simulink model "ADCS_Outline"  (R2019a)
settings: Solver=VariableStepAuto  StartTime=0.0  StopTime=duration  MaxStep=step
InitFcn:
  | SC_ODIN_INITIALIZATION
values from neighbouring files (symbols this model uses):
  A = [ v(1) v(4) v(5) v(7);        v(4) v(2) v(6) v(8);        v(5) v(6) v(3) v(9);        v(7) v(8) v(9) v(10) ]    [MagnetometerCalibration.m]    (also in SC_ODIN_INITIALIZATION.m = 0.06; test.m = asin(sin(N)/sin(n)*sin(a)))
  Amag = [0.910186583854  -0.00959593267728  0.00343590491018; -0.00959593267728  1.05471221352  0.0559849466324; 0.00343590491018  0.0559849466324  1.05528532305]    [MagnetometerBias.mat]    (also in MagnetometerCalibration.m = evecs/scale*evecs')
  argentina = [1612.36;-4182.16;-4522.83]    [SC_ODIN_INITIALIZATION.m]
  As = 0.2*0.3    (= 0.06)    [SC_ODIN_INITIALIZATION.m]
  b_mag = block.InputPort(3).Data    [MagnetometerCalibration.m]    (also in SC_ODIN_INITIALIZATION.m = [10;-15.5;-12.2]*1e-6)
  bmag = [1.00003671399e-05 -1.55007781395e-05 -1.22009762149e-05]    [MagnetometerBias.mat]    (also in MagnetometerCalibration.m = centerE)
  breakpoints = data(:,1)    [SC_ODIN_INITIALIZATION.m]
  c = 2.99792458e8    (= 299792458)    [SC_ODIN_INITIALIZATION.m]
  C_I = [0.045 0.0009 -0.00007;        0.0009 0.045 -0.00003;        -0.00007 -0.00003 0.009]    [SC_ODIN_INITIALIZATION.m]
  Cd = 2.0    (= 2)    [SC_ODIN_INITIALIZATION.m]
  controller_sample_rate = 0.5    [SC_ODIN_INITIALIZATION.m]
  D = [ 2 * x,            2 * y,            2 * z,            1 + 0 * x ]    [MagnetometerCalibration.m]    (also in SC_ODIN_INITIALIZATION.m = 0.01*[1;1;1])
  datapx = data(:,2)    [SC_ODIN_INITIALIZATION.m]
  datapy = data(:,3)    [SC_ODIN_INITIALIZATION.m]
  datapz = data(:,4)    [SC_ODIN_INITIALIZATION.m]
  datavx = data(:,5)    [SC_ODIN_INITIALIZATION.m]
  datavy = data(:,6)    [SC_ODIN_INITIALIZATION.m]
  datavz = data(:,7)    [SC_ODIN_INITIALIZATION.m]
  DCM_BT0 = eye(3)    [SC_ODIN_INITIALIZATION.m]
  G = 6.67408e-11    [SC_ODIN_INITIALIZATION.m]
  ground = [1266.06;-4295.81;4526.14]    [SC_ODIN_INITIALIZATION.m]
  I = [Ixx -Ixy -Ixz;      -Ixy Iyy -Iyz;      -Ixz -Iyz Izz]    [SC_ODIN_INITIALIZATION.m]
  invA_mag = block.InputPort(2).Data    [MagnetometerCalibration.m]    (also in SC_ODIN_INITIALIZATION.m = inv(Ellrot/scale*Ellrot'))
  JD_0 = start_day+start_fraction    [SC_ODIN_INITIALIZATION.m]
  Ks = 1367    [SC_ODIN_INITIALIZATION.m]
  L = [0.0000812 -0.0022136 -0.0225868]    [SC_ODIN_INITIALIZATION.m]
  Ls = 0.01*[-3; 3; 5]    [SC_ODIN_INITIALIZATION.m]
  M = 5.9722e24    (= 5.9722e+24)    [SC_ODIN_INITIALIZATION.m]    (also in visualisation.m = uicontrol('Style','text','String',{''},'Position',[710 100+2)
  magnetorquer_tau = 0.02    [SC_ODIN_INITIALIZATION.m]
  magnetorquer_x_saturation = 0.24    [SC_ODIN_INITIALIZATION.m]
  magnetorquer_y_saturation = 0.24    [SC_ODIN_INITIALIZATION.m]
  magnetorquer_z_saturation = 0.13    [SC_ODIN_INITIALIZATION.m]
  namibia = [5659.26;1238.85;-2659.2]    [SC_ODIN_INITIALIZATION.m]
  q = 0.6    [SC_ODIN_INITIALIZATION.m]
  radii = radii .* sgns    [MagnetometerCalibration.m]    (also in SC_ODIN_INITIALIZATION.m = [1;0.9;1.1])
  W0 = [1;0;1-1/240].*pi()/180    [SC_ODIN_INITIALIZATION.m]
  wheel_saturation = 0.23e-3    (= 0.00023)    [SC_ODIN_INITIALIZATION.m]
  wheel_tau = 2    [SC_ODIN_INITIALIZATION.m]
undefined symbols (not defined in the file or in its folder): DiscIntNeverNeededParam, nut80, sun_sensors
libraries: dspmathops x94, vrlib x70, dspsrcs4 x21, realtime_pacer_lib x1, dspsolvers x1, dspinverses x1
(part 5 of 6)

== matlab function ADCS_Outline/Sun/MATLAB Function2 ==
  data: ddpsi input; ddeps input; reci input; nut80 input; rteme output; ttt input
% ----------------------------------------------------------------------------
%
%                           function eci2teme
%
%  this function transforms a vector from the mean equator mean equinox (j2000) 
%    system (eci), to the true equator mean equinox (teme) system.
%
%  author        : david vallado                  719-573-2600   30 oct 2017
%
%  inputs          description                    range / units
%    reci        - position vector eci            km
%    veci        - velocity vector eci            km/s
%    aeci        - acceleration vector eci        km/s2
%    ttt         - julian centuries of tt         centuries
%    ddpsi       - delta psi correction to gcrf   rad
%    ddeps       - delta eps correction to gcrf   rad
%
%  outputs       :
%    rteme       - position vector of date
%                    true equator, mean equinox   km
%    vteme       - velocity vector of date
%                    true equator, mean equinox   km/s
%    ateme       - acceleration vector of date
%                    true equator, mean equinox   km/s2
%
%  locals        :
%    prec        - matrix for eci - mod
%    nutteme     - matrix for mod - teme - an approximation for nutation
%    eqe         - rotation for equation of equinoxes (geometric terms only)
%    tm          - combined matrix for teme2eci
%
%  coupling      :
%   precess      - rotation for precession        eci - mod
%   nutation     - rotation for nutation          eci - tod
%
%  references    :
%    vallado       2013, 231-233
%
% [reci, veci, aeci] = teme2eci  ( rteme, vteme, ateme, ttt, ddpsi, ddeps);
% ----------------------------------------------------------------------------

function rteme  = eci2teme  (ddpsi, ddeps, reci, nut80, ttt)

        prec = zeros(3,3);
        [prec,psia, wa, ea, xa] = precess ( ttt );

        [deltapsi, trueeps, meaneps, omega, nut] = nutation  (ttt, ddpsi, ddeps, nut80);
        
        % ------------------------ find eqeg ----------------------
        % rotate teme through just geometric terms 
        eqeg = deltapsi* cos(meaneps);

        eqeg = rem (eqeg, 2.0*pi);

        eqe = zeros(3,3);
        eqe(1,1) =  cos(eqeg);
        eqe(1,2) =  sin(eqeg);
        eqe(1,3) =  0.0;
        eqe(2,1) = -sin(eqeg);
        eqe(2,2) =  cos(eqeg);
        eqe(2,3) =  0.0;
        eqe(3,1) =  0.0;
        eqe(3,2) =  0.0;
        eqe(3,3) =  1.0;

        tm = eqe * nut' * prec';
        
        rteme = tm * reci;
        

%�
% ----------------------------------------------------------------------------
%
%                           function precess
%
%  this function calulates the transformation matrix that accounts for the effects
%    of precession. both the 1980 and 2000 theories are handled. note that the 
%    required parameters differ a little. 
%
%  author        : david vallado                  719-573-2600   25 jun 2002
%
%  revisions
%    vallado     - consolidate with iau 2000                     14 feb 2005
%
%  inputs          description                    range / units
%    ttt         - julian centuries of tt
%    opt         - method option                  '01', '02', '96', '80'
%
%  outputs       :
%    prec        - transformation matrix for mod - j2000 (80 only)
%    psia        - cannonical precession angle    rad    (00 only)
%    wa          - cannonical precession angle    rad    (00 only)
%    ea          - cannonical precession angle    rad    (00 only)
%    xa          - cannonical precession angle    rad    (00 only)
%
%  locals        :
%    ttt2        - ttt squared
%    ttt3        - ttt cubed
%    zeta        - precession angle               rad
%    z           - precession angle               rad
%    theta       - precession angle               rad
%    oblo        - obliquity value at j2000 epoch "%
%
%  coupling      :
%    none        -
%
%  references    :
%    vallado       2004, 214-216, 219-221
%
% [prec,psia,wa,ea,xa] = precess ( ttt, opt );
% ----------------------------------------------------------------------------

function [prec,psia,wa,ea,xa] = precess ( ttt );

       % sethelp;
        
        % " to rad
        convrt = pi / (180.0*3600.0);
        ttt2= ttt * ttt;
        ttt3= ttt2 * ttt;

        % ------------------- fk4 b1950 precession angles --------------------
%         if (opt == '50')
% 
%             % ---- Seidelmann pg 107             
%             % for these calls, ttt will come in with the current jd
% %            t1= 0.0; %(ttt - 2433282.42345905)/365242.198782;  % set start as B1850, 0.0 to simplify
% %            t2= (ttt - 2396758.203)/365242.198782;  % uses B1850
% %            ttt = t2 - t1;
% %            ttt2 = ttt * ttt;
% %            ttt3 = ttt * ttt2;
% %            fprintf(1,'50prec %15.9f  \n',ttt);
%             % exp supp 61 pg 38
% %            psia = 50.3708 + 0.0050 * ttt;
% %            wa = 0.0;
% %            ea = 0.0;
% %            xa = 0.1247 - 0.0188 * ttt;
% %            zeta =  (23035.545 + 139.720*t1 + 0.060 *t1*t1)*ttt + (30.240-0.270*t1)*ttt2 + 17.995*ttt3; % "
% %            theta=  (20051.12 - 85.29*t1 - 0.37 *t1*t1)*ttt + (-42.65-0.37*t1)*ttt2 - 41.80*ttt3;
% %            z    =  (23035.545 + 139.720*t1 + 0.060 *t1*t1)*ttt + (109.480+0.390*t1)*ttt2 + 18.325*ttt3;
% 
%             % ---- Newcomb Exp Supp 61 approach, but see GTDS pg 3-17
%             % Exp Supp 61 says use 1900? but gtds says use 1950. 
%             % for these calls, ttt will come in with the current jd
%             t1= 0.0; %(ttt - 2415020.31352)/36524.2198782;  % set start as B1900, 0.0 to simplify
% %            t2= (ttt - 2415020.31352)/36525;  % uses B1900   
%             t2= (ttt - 2433282.42345905)/36525;  % uses B1950  
% %            ttt = t2 - t1;
% %            ttt2 = ttt * ttt;
% %            ttt3 = ttt * ttt2;
%             % exp supp 61 pg 38
%             psia = 50.3708 + 0.0050 * ttt;
%             wa = 0.0; % not sure which one is which...
%             ea = 84428.26 -   46.845*ttt - 0.00059*ttt2 + 0.00181*ttt3;
%             xa = 0.1247 - 0.0188 * ttt;
%            fprintf(1,'50prec %15.9f  \n',ttt);
%            % seems like Exp supp 61 is ok with 1900 as epoch, and Seidlemann is ok with listed measr,  
% %            zeta =  (2304.25 + 1.396*t1)*ttt + 0.302*ttt2 + 0.018*ttt3; % "
% %            theta=  (2004.682 - 0.853*t1)*ttt -0.426*ttt2 - 0.042*ttt3;
% %            z    =  (2304.25 + 1.396*t1)*ttt + 1.093*ttt2 + 0.018*ttt3;
%             % GTDS pg 3-17 using days from 1950 - avoids long rpecession
%             % constants...
%             zeta =  2304.9969*ttt + 0.302*ttt2 + 0.01808*ttt3; % "
%             theta=  2004.2980*ttt -0.425936*ttt2 - 0.0416*ttt3;
%             z    =  2304.9969*ttt + 1.092999*ttt2 + 0.0192*ttt3;
%             
% 
%             % tp-008 36-45
%             % ttt is tropical centruies from 1950 36524.22 days
%             prec = zeros(3,3);
%             prec(1,1) =  1.0 - 2.9696e-4 * ttt2 - 1.3e-7 * ttt3;
%             prec(1,2) =  2.234941e-2 * ttt + 6.76e-6 * ttt2 - 2.21e-6 * ttt3;
%             prec(1,3) =  9.7169e-3 * ttt - 2.07e-6 * ttt2 - 9.6e-7 * ttt3;
%             prec(2,1) =  -prec(1,2);
%             prec(2,2) =  1.0 - 2.4975e-4 * ttt2 - 1.5e-7 * ttt3;
%             prec(2,3) =  - 1.0858e-4 * ttt2;
%             prec(3,1) =  -prec(1,3);
%             prec(3,2) =  prec(2,3);
%             prec(3,3) =  1.0 - 4.721e-5 * ttt2;
%  
%             
%            % pass these back out for testing
%            psia = zeta;
%            wa = theta;
%            ea = z;
%         % ------------------- iau 76 precession angles --------------------
%         else
%           if (opt == '80')
%     fprintf(1,'80prec %15.9f  \n',ttt);
            psia =             5038.7784*ttt - 1.07259*ttt2 - 0.001147*ttt3; % "
            wa   = 84381.448                 + 0.05127*ttt2 - 0.007726*ttt3;
            ea   = 84381.448 -   46.8150*ttt - 0.00059*ttt2 + 0.001813*ttt3;
            xa   =               10.5526*ttt - 2.38064*ttt2 - 0.001125*ttt3;
            zeta =             2306.2181*ttt + 0.30188*ttt2 + 0.017998*ttt3; % "
            theta=             2004.3109*ttt - 0.42665*ttt2 - 0.041833*ttt3;
            z    =             2306.2181*ttt + 1.09468*ttt2 + 0.018203*ttt3;
          % ------------------ iau 03 precession angles -------------------
%           else
%             oblo =  84381.406; % "
%             psia =  (((( -0.0000000951 * ttt + 0.000132851 ) * ttt - 0.00114045 ) * ttt - 1.0790069 ) * ttt + 5038.481507 ) * ttt; % "
%             wa   =  ((((  0.0000003337 * ttt - 0.000000467 ) * ttt - 0.00772503 ) * ttt + 0.0512623 ) * ttt -    0.025754 ) * ttt + oblo;
%             ea   =  (((( -0.0000000434 * ttt - 0.000000576 ) * ttt + 0.00200340 ) * ttt - 0.0001831 ) * ttt -   46.836769 ) * ttt + oblo;
%             xa   =  (((( - 0.0000000560 * ttt + 0.000170663 ) * ttt - 0.00121197 ) * ttt - 2.3814292 ) * ttt +   10.556403 ) * ttt;
% 
%             zeta =  (((( - 0.0000003173 * ttt - 0.000005971 ) * ttt + 0.01801828 ) * ttt + 0.2988499 ) * ttt + 2306.083227 ) * ttt + 2.650545; % "
%             theta=  (((( - 0.0000001274 * ttt - 0.000007089 ) * ttt - 0.04182264 ) * ttt - 0.4294934 ) * ttt + 2004.191903 ) * ttt;
%             z    =  ((((   0.0000002904 * ttt - 0.000028596 ) * ttt + 0.01826837 ) * ttt + 1.0927348 ) * ttt + 2306.077181 ) * ttt - 2.650545;
%           end;
%         end;
        
        % convert units to rad
        psia = psia  * convrt; % rad
        wa   = wa    * convrt;
        ea   = ea    * convrt;
        xa   = xa    * convrt;
        zeta = zeta  * convrt; 
        theta= theta * convrt;
        z    = z     * convrt;
%iauhelp='y';         
%fprintf(1,'pr %11.7f  %11.7f  %11.7fdeg \n',zeta*180/pi,theta*180/pi,z*180/pi );
%         if (iauhelp == 'y')
%             fprintf(1,'pr %11.7f  %11.7f  %11.7f %11.7fdeg \n',psia*180/pi,wa*180/pi,ea*180/pi,xa*180/pi );
%             fprintf(1,'pr %11.7f  %11.7f  %11.7fdeg \n',zeta*180/pi,theta*180/pi,z*180/pi );
%         end;
% 
%         if (strcmp(opt,'80')==1) % || (strcmp(opt,'50') == 1)
            coszeta  = cos(zeta);
            sinzeta  = sin(zeta);
            costheta = cos(theta);
            sintheta = sin(theta);
            cosz     = cos(z);
            sinz     = sin(z);

            % ----------------- form matrix  mod to j2000 -----------------
            prec = zeros(3,3);
            prec(1,1) =  coszeta * costheta * cosz - sinzeta * sinz;
            prec(1,2) =  coszeta * costheta * sinz + sinzeta * cosz;
            prec(1,3) =  coszeta * sintheta;
            prec(2,1) = -sinzeta * costheta * cosz - coszeta * sinz;
            prec(2,2) = -sinzeta * costheta * sinz + coszeta * cosz;
            prec(2,3) = -sinzeta * sintheta;
            prec(3,1) = -sintheta * cosz;
            prec(3,2) = -sintheta * sinz;
            prec(3,3) =  costheta;

            % ----------------- do rotations instead ----------------------
            % p1 = rot3mat( z );
            % p2 = rot2mat( -theta );
            % p3 = rot3mat( zeta );
            % prec = p3*p2*p1;
%         elseif (strcmp(opt,'50') ~= 1)
%             oblo = oblo * convrt; % " to rad
%             a4  = rot3mat(-xa);
%             a5  = rot1mat(wa);
%             a6  = rot3mat(psia);
%             a7  = rot1mat(-oblo);
%             prec = a7*a6*a5*a4;
%            % prec = zeros(3);
%         end;



% ----------------------------------------------------------------------------
%
%                           function nutation
%
%  this function calulates the transformation matrix that accounts for the
%    effects of nutation.
%
%  author        : david vallado                  719-573-2600   27 jun 2002
%
%  revisions
%    vallado     - consolidate with iau 2000                     14 feb 2005
%
%  inputs          description                    range / units
%    ttt         - julian centuries of tt
%    ddpsi       - delta psi correction to gcrf   rad
%    ddeps       - delta eps correction to gcrf   rad
%
%  outputs       :
%    deltapsi    - nutation angle                 rad
%    trueeps     - true obliquity of the ecliptic rad
%    meaneps     - mean obliquity of the ecliptic rad
%    omega       -                                rad
%    nut         - transformation matrix for tod - mod
%
%  locals        :
%    iar80       - integers for fk5 1980
%    rar80       - reals for fk5 1980
%    ttt2        - ttt squared
%    ttt3        - ttt cubed
%    l           -                                rad
%    ll          -                                rad
%    f           -                                rad
%    d           -                                rad
%    deltaeps    - change in obliquity            rad
%
%  coupling      :
%    fundarg     - find fundamental arguments
%
%  references    :
%    vallado       2013, 224-226
%
% [deltapsi, trueeps, meaneps, omega,nut] = nutation  (ttt, ddpsi, ddeps );
% ----------------------------------------------------------------------------

function [deltapsi, trueeps, meaneps, omega,nut] = nutation  (ttt, ddpsi, ddeps , nut80);

        deg2rad = pi/180.0;

        [iar80,rar80] =  iau80in(nut80);  % coeff in deg

        % ---- determine coefficients for iau 1980 nutation theory ----
        ttt2= ttt*ttt;
        ttt3= ttt2*ttt;

        meaneps = -46.8150 *ttt - 0.00059 *ttt2 + 0.001813 *ttt3 + 84381.448;
        meaneps = rem( meaneps/3600.0, 360.0 );
        meaneps = meaneps * deg2rad;

        [ l, l1, f, d, omega, ...
          lonmer, lonven, lonear, lonmar, lonjup, lonsat, lonurn, lonnep, precrate ...
        ] = fundarg( ttt, '80' );
%fprintf(1,'nut del arg %11.7f  %11.7f  %11.7f  %11.7f  %11.7f  \n',l*180/pi,l1*180/pi,f*180/pi,d*180/pi,omega*180/pi );

        deltapsi= 0.0;
        deltaeps= 0.0;
        for i= 106:-1: 1
            tempval= iar80(i,1)*l + iar80(i,2)*l1 + iar80(i,3)*f + ...
                     iar80(i,4)*d + iar80(i,5)*omega;
            deltapsi= deltapsi + (rar80(i,1)+rar80(i,2)*ttt) * sin( tempval );
            deltaeps= deltaeps + (rar80(i,3)+rar80(i,4)*ttt) * cos( tempval );
        end

        % --------------- find nutation parameters --------------------
        deltapsi = rem( deltapsi + ddpsi, 2.0 * pi );
        deltaeps = rem( deltaeps + ddeps, 2.0 * pi );
        trueeps  = meaneps + deltaeps;

%fprintf(1,'meaneps %11.7f dp  %11.7f de  %11.7f te  %11.7f  ttt  %11.7f \n',meaneps*180/pi,deltapsi*180/pi,deltaeps*180/pi,trueeps*180/pi, ttt );

        cospsi  = cos(deltapsi);
        sinpsi  = sin(deltapsi);
        coseps  = cos(meaneps);
        sineps  = sin(meaneps);
        costrueeps = cos(trueeps);
        sintrueeps = sin(trueeps);
        
        nut = zeros(3,3);
        nut(1,1) =  cospsi;
        nut(1,2) =  costrueeps * sinpsi;
        nut(1,3) =  sintrueeps * sinpsi;
        nut(2,1) = -coseps * sinpsi;
        nut(2,2) =  costrueeps * coseps * cospsi + sintrueeps * sineps;
        nut(2,3) =  sintrueeps * coseps * cospsi - sineps * costrueeps;
        nut(3,1) = -sineps * sinpsi;
        nut(3,2) =  costrueeps * sineps * cospsi - sintrueeps * coseps;
        nut(3,3) =  sintrueeps * sineps * cospsi + costrueeps * coseps;

      %   n1 = rot1mat( trueeps );
      %   n2 = rot3mat( deltapsi );
      %   n3 = rot1mat( -meaneps );
      %   nut = n3*n2*n1

%�
% ----------------------------------------------------------------------------
%
%                           function fundarg
%
%  this function calulates the delauany variables and planetary values for
%  several theories.
%
%  author        : david vallado                  719-573-2600   16 jul 2004
%
%  revisions
%    vallado     - consolidate with iau 2000                     14 feb 2005
%
%  inputs          description                    range / units
%    ttt         - julian centuries of tt
%    opt         - method option                  '10', '02', '96', '80'
%
%  outputs       :
%    l           - delaunay element               rad
%    ll          - delaunay element               rad
%    f           - delaunay element               rad
%    d           - delaunay element               rad
%    omega       - delaunay element               rad
%    planetary longitudes                         rad
%
%  locals        :
%    ttt2,ttt3,  - powers of ttt
%
%  coupling      :
%    none        -
%
%  references    :
%    vallado       2004, 212-214
%
% [ l, l1, f, d, omega, ...
%   lonmer, lonven, lonear, lonmar, lonjup, lonsat, lonurn, lonnep, precrate ...
% ] = fundarg( ttt, opt );
% ----------------------------------------------------------------------------

function [ l, l1, f, d, omega, ...
           lonmer, lonven, lonear, lonmar, lonjup, lonsat, lonurn, lonnep, precrate ...
         ] = fundarg( ttt, opt )

        %sethelp;

        deg2rad = pi/180.0;

        % ---- determine coefficients for iau 2000 nutation theory ----
        ttt2 = ttt*ttt;
        ttt3 = ttt2*ttt;
        ttt4 = ttt2*ttt2;

        % ---- iau 2010 theory
        if opt == '10'
            % ------ form the delaunay fundamental arguments in deg
            l    =  134.96340251  + ( 1717915923.2178 *ttt + ...
                     31.8792 *ttt2 + 0.051635 *ttt3 - 0.00024470 *ttt4 ) / 3600.0;
            l1   =  357.52910918  + (  129596581.0481 *ttt - ...
                      0.5532 *ttt2 - 0.000136 *ttt3 - 0.00001149*ttt4 )  / 3600.0;
            f    =   93.27209062  + ( 1739527262.8478 *ttt - ...
                     12.7512 *ttt2 + 0.001037 *ttt3 + 0.00000417*ttt4 )  / 3600.0;
            d    =  297.85019547  + ( 1602961601.2090 *ttt - ...
                      6.3706 *ttt2 + 0.006593 *ttt3 - 0.00003169*ttt4 )  / 3600.0;
            omega=  125.04455501  + (   -6962890.5431 *ttt + ...
                      7.4722 *ttt2 + 0.007702 *ttt3 - 0.00005939*ttt4 )  / 3600.0;

            % ------ form the planetary arguments in deg
            lonmer  = 252.250905494  + 149472.6746358  *ttt;
            lonven  = 181.979800853  +  58517.8156748  *ttt;
            lonear  = 100.466448494  +  35999.3728521  *ttt;
            lonmar  = 355.433274605  +  19140.299314   *ttt;
            lonjup  =  34.351483900  +   3034.90567464 *ttt;
            lonsat  =  50.0774713998 +   1222.11379404 *ttt;
            lonurn  = 314.055005137  +    428.466998313*ttt;
            lonnep  = 304.348665499  +    218.486200208*ttt;
            precrate=   1.39697137214*ttt + 0.0003086*ttt2;
         end;

        % ---- iau 2000b theory
        if opt == '02'
            % ------ form the delaunay fundamental arguments in deg
            l    =  134.96340251  + ( 1717915923.2178 *ttt ) / 3600.0;
            l1   =  357.52910918  + (  129596581.0481 *ttt ) / 3600.0;
            f    =   93.27209062  + ( 1739527262.8478 *ttt ) / 3600.0;
            d    =  297.85019547  + ( 1602961601.2090 *ttt ) / 3600.0;
            omega=  125.04455501  + (   -6962890.5431 *ttt ) / 3600.0;

            % ------ form the planetary arguments in deg
            lonmer  = 0.0;
            lonven  = 0.0;
            lonear  = 0.0;
            lonmar  = 0.0;
            lonjup  = 0.0;
            lonsat  = 0.0;
            lonurn  = 0.0;
            lonnep  = 0.0;
            precrate= 0.0;
         end;   

        % ---- iau 1996 theory
        if opt == '96'
            l    =  134.96340251  + ( 1717915923.2178 *ttt + ...
                     31.8792 *ttt2 + 0.051635 *ttt3 - 0.00024470 *ttt4 ) / 3600.0;
            l1   =  357.52910918  + (  129596581.0481 *ttt - ...
                      0.5532 *ttt2 - 0.000136 *ttt3 - 0.00001149*ttt4 )  / 3600.0;
            f    =   93.27209062  + ( 1739527262.8478 *ttt - ...
                     12.7512 *ttt2 + 0.001037 *ttt3 + 0.00000417*ttt4 )  / 3600.0;
            d    =  297.85019547  + ( 1602961601.2090 *ttt - ...
                      6.3706 *ttt2 + 0.006593 *ttt3 - 0.00003169*ttt4 )  / 3600.0;
            omega=  125.04455501  + (   -6962890.2665 *ttt + ...
                      7.4722 *ttt2 + 0.007702 *ttt3 - 0.00005939*ttt4 )  / 3600.0;
            % ------ form the planetary arguments in deg
            lonmer  = 0.0;
            lonven  = 181.979800853  +  58517.8156748  *ttt;   % deg
            lonear  = 100.466448494  +  35999.3728521  *ttt;
            lonmar  = 355.433274605  +  19140.299314   *ttt;
            lonjup  =  34.351483900  +   3034.90567464 *ttt;
            lonsat  =  50.0774713998 +   1222.11379404 *ttt;
            lonurn  = 0.0;
            lonnep  = 0.0;
            precrate=   1.39697137214*ttt + 0.0003086*ttt2;
         end;   

         % ---- iau 1980 theory
        if opt == '80'
            l = ((((0.064) * ttt + 31.310) * ttt + 1717915922.6330) * ttt) / 3600.0 + 134.96298139;
    		l1 = ((((-0.012) * ttt - 0.577) * ttt + 129596581.2240) * ttt) / 3600.0 + 357.52772333;
    		f = ((((0.011) * ttt - 13.257) * ttt + 1739527263.1370) * ttt) / 3600.0 + 93.27191028;
	    	d = ((((0.019) * ttt - 6.891) * ttt + 1602961601.3280) * ttt) / 3600.0 + 297.85036306;
    		omega = ((((0.008) * ttt + 7.455) * ttt - 6962890.5390) * ttt) / 3600.0 + 125.04452222;
                  
            % ------ form the planetary arguments in deg
            lonmer  = 252.3 + 149472.0 *ttt;
            lonven  = 179.9 +  58517.8 *ttt;   % deg
            lonear  =  98.4 +  35999.4 *ttt;
            lonmar  = 353.3 +  19140.3 *ttt;
            lonjup  =  32.3 +   3034.9 *ttt;
            lonsat  =  48.0 +   1222.1 *ttt;
            lonurn  =   0.0;
            lonnep  =   0.0;
            precrate=   0.0;
         end;   

        % ---- convert units to rad
        l    = rem( l,360.0  )     * deg2rad; % rad
        l1   = rem( l1,360.0  )    * deg2rad;
        f    = rem( f,360.0  )     * deg2rad;
        d    = rem( d,360.0  )     * deg2rad;
        omega= rem( omega,360.0  ) * deg2rad;

        lonmer= rem( lonmer,360.0 ) * deg2rad;  % rad
        lonven= rem( lonven,360.0 ) * deg2rad;
        lonear= rem( lonear,360.0 ) * deg2rad;
        lonmar= rem( lonmar,360.0 ) * deg2rad;
        lonjup= rem( lonjup,360.0 ) * deg2rad;
        lonsat= rem( lonsat,360.0 ) * deg2rad;
        lonurn= rem( lonurn,360.0 ) * deg2rad;
        lonnep= rem( lonnep,360.0 ) * deg2rad;
        precrate= rem( precrate,360.0 ) * deg2rad;
%iauhelp='y';
%         if iauhelp == 'y'
%             fprintf(1,'fa %11.7f  %11.7f  %11.7f  %11.7f  %11.7f deg \n',l*180/pi,l1*180/pi,f*180/pi,d*180/pi,omega*180/pi );
%             fprintf(1,'fa %11.7f  %11.7f  %11.7f  %11.7f deg \n',lonmer*180/pi,lonven*180/pi,lonear*180/pi,lonmar*180/pi );
%             fprintf(1,'fa %11.7f  %11.7f  %11.7f  %11.7f deg \n',lonjup*180/pi,lonsat*180/pi,lonurn*180/pi,lonnep*180/pi );
%             fprintf(1,'fa %11.7f  \n',precrate*180/pi );
%           end;

function [iar80,rar80] = iau80in(nut80);

       % ------------------------  implementation   -------------------
       % 0.0001" to rad
       convrt= 0.0001 * pi / (180*3600.0);

       %load nut80.dat;

       iar80 = nut80(:,1:5);
       rar80 = nut80(:,6:9);

       for i=1:106
           for j=1:4
               rar80(i,j)= rar80(i,j) * convrt;
           end
       end

== matlab function ADCS_Outline/S//C Kinematics/Skewed/MATLAB Function ==
  data: u input; y output
function y = fcn(u)
y = [0 -u(3) u(2); ...
     u(3) 0 -u(1); ...
    -u(2) u(1) 0];

== matlab function ADCS_Outline/Momentum Control/Momentum Bias/Rotation/     ==
  data: qa input; q output; qb input
function q = Quatmultiply(qa,qb)

q4 = qa(4)*qb(4) - qa(1)*qb(1) - qa(2)*qb(2) - qa(3)*qb(3);
q1 = qa(4)*qb(1) + qa(1)*qb(4) + qa(2)*qb(3) - qa(3)*qb(2);
q2 = qa(4)*qb(2) - qa(1)*qb(3) + qa(2)*qb(4) + qa(3)*qb(1);
q3 = qa(4)*qb(3) + qa(1)*qb(2) - qa(2)*qb(1) + qa(3)*qb(4);

q = [q1 q2 q3 q4];

== matlab function ADCS_Outline/Reaction Wheels/MATLAB Function ==
  data: Ti input; Tw output; Lw input
function Tw = saturation_rw(Ti,Lw)

sat1 = abs(Lw(1))/1.77e-3;
sat2 = abs(Lw(2))/1.77e-3;
sat3 = abs(Lw(3))/1.77e-3;

if sat1>1 && Ti(1)*Lw(1)>0
    T1 = 0;
else 
    T1 = Ti(1);
end

if sat2>1 && Ti(2)*Lw(2)>0
    T2 = 0;
else 
    T2 = Ti(2);
end

if sat3>1 && Ti(3)*Lw(3)>0
    T3 = 0;
else 
    T3 = Ti(3);
end

Tw = [T1;T2;T3];

== matlab function ADCS_Outline/Toolbox/No Control fast STK attitude recoding/Mode Selector ==
  data: P input; A input; N input; G input; Mode output
function Mode  = Selector(P,A,N,G)

        if dot(P,A)/(norm(P)*norm(A)) > 0.96 %In range of Argentina
           Mode = 3; %Imaging Argentina
        elseif dot(P,N)/(norm(P)*norm(N)) > 0.96 %In range of Namibia
           Mode = 4; %Imaging Namibia 
        elseif dot(P,G)/(norm(P)*norm(G)) > 0.91 %In range of ground
           Mode = 2; %Ground
        else
           Mode = 5; %Nadir  
        end

end

== matlab function ADCS_Outline/VISUALISATION/MATLAB Function2 ==
  data: DCM input; yaw output; pitch output; roll output
function [yaw, pitch, roll] = DCM2euler(DCM)

yaw = atan2(DCM(2,1),DCM(1,1));
pitch = asin(min(1, max(-1, -DCM(3,1))));
roll = atan2(DCM(3,2),DCM(3,3));

end

== matlab function ADCS_Outline/Momentum Control/Momentum Bias/Rotation/    1 ==
  data: qa input; q output; qb input
function q = Quatmultiply(qa,qb)

q4 = qa(4)*qb(4) - qa(1)*qb(1) - qa(2)*qb(2) - qa(3)*qb(3);
q1 = qa(4)*qb(1) + qa(1)*qb(4) + qa(2)*qb(3) - qa(3)*qb(2);
q2 = qa(4)*qb(2) - qa(1)*qb(3) + qa(2)*qb(4) + qa(3)*qb(1);
q3 = qa(4)*qb(3) + qa(1)*qb(2) - qa(2)*qb(1) + qa(3)*qb(4);

q = [q1 q2 q3 q4];

== matlab function ADCS_Outline/Toolbox/No Control fast STK attitude recoding/Perfect DCM1/Mode Selection ==
  data: Mode input; DCM_EF input; DCM_FS input; DCM_ETarget output; DCM_FG input; DCM_FA input; DCM_FN input; DCM_FZ input
function DCM_ETarget   = fcn(Mode,DCM_EF,DCM_FS,DCM_FG, DCM_FA, DCM_FN, DCM_FZ)

switch Mode
    case 1
      DCM_ETarget = DCM_EF*DCM_FS;
    case 2
      DCM_ETarget = DCM_EF*DCM_FG;
    case 3
      DCM_ETarget = DCM_EF*DCM_FA;
    case 4
      DCM_ETarget = DCM_EF*DCM_FN;
    case 5
      DCM_ETarget = DCM_EF*DCM_FZ;
    otherwise 
      DCM_ETarget = eye(3);
end

== matlab function ADCS_Outline/Momentum Control/Switch ==
  data: CM output; Mode input; Eclipse input; Bdot input; M output; Nominal input
function [CM,M] = fcn(Mode,Eclipse,Bdot,Nominal)

persistent pause

switch Mode
    
    case 2 %ground
        M = [0;0;0];
        CM = [0;0;0];
    case 3 %imagingA
        M = [0;0;0];
        CM = [0;0;0];
    case 4 %imgaing N
        M = [0;0;0];
        CM = [0;0;0];
    case 6 %detumbling
        M = Bdot;
        CM = Bdot;
    case 7 %OFF
        M = [0;0;0];
        CM = [0;0;0];
    case 8 %calibration
        M = [0;0;0];
        CM = [0;0;0];
    otherwise
        M = Nominal;
        CM = Nominal;
        
end

if isempty(pause)
    pause = 1;
elseif pause >=1%stops magnetorquers to get a reading
    pause = 0;
    M = [0;0;0];
    CM = Nominal;
elseif ismember(Mode,[1 5 6])
    pause = pause + 1;
end

if (Eclipse == 1) && (Mode~=6)
     M = [0;0;0];
    CM = [0;0;0];  
end

if Mode==6
    CM = Bdot;
end

== matlab function ADCS_Outline/STK Attitude Recording/DCM to q ==
  data: dcm_inv input; q output
function q = fcn(dcm_inv)

dcm = transpose(dcm_inv);
tr = trace(dcm);

if (tr > 0) 
  S = sqrt(tr+1.0) * 2; % S=4*qw 
  qw = 0.25 * S;
  qx = (dcm(3,2) - dcm(2,3)) / S;
  qy = (dcm(1,3) - dcm(3,1)) / S; 
  qz = (dcm(2,1) - dcm(1,2)) / S; 
elseif ((dcm(1,1) > dcm(2,2)) && (dcm(1,1) > dcm(3,3))) 
  S = sqrt(1.0 + dcm(1,1) - dcm(2,2) - dcm(3,3)) * 2; % S=4*qx 
  qw = (dcm(3,2) - dcm(2,3)) / S;
  qx = 0.25 * S;
  qy = (dcm(1,2) + dcm(2,1)) / S; 
  qz = (dcm(1,3) + dcm(3,1)) / S; 
elseif (dcm(2,2) > dcm(3,3)) 
  S = sqrt(1.0 + dcm(2,2) - dcm(1,1) - dcm(3,3)) * 2; % S=4*qy
  qw = (dcm(1,3) - dcm(3,1)) / S;
  qx = (dcm(1,2) + dcm(2,1)) / S; 
  qy = 0.25 * S;
  qz = (dcm(2,3) + dcm(3,2)) / S; 
 else  
  S = sqrt(1.0 + dcm(3,3) - dcm(1,1) - dcm(2,2)) * 2; % S=4*qz
  qw = (dcm(2,1) - dcm(1,2)) / S;
  qx = (dcm(1,3) + dcm(3,1)) / S;
  qy = (dcm(2,3) + dcm(3,2)) / S;
  qz = 0.25 * S;
end
q = [qx;qy;qz;qw];

== matlab function ADCS_Outline/VISUALISATION/MATLAB Function1 ==
  data: DCM input; yaw output; pitch output; roll output
function [yaw, pitch, roll] = DCM2euler(DCM)

yaw = atan2(DCM(2,1),DCM(1,1));
pitch = asin(min(1, max(-1, -DCM(3,1))));
roll = atan2(DCM(3,2),DCM(3,3));

end

== matlab function ADCS_Outline/Toolbox/Angle between vectors ==
  data: u input; y output; v input
function y = fcn(u,v)

y = acos(dot(u,v)/(norm(u)*norm(v)))*180/pi;

== matlab function ADCS_Outline/Reaction Wheels Control/MATLAB Function ==
  data: Lw input; Ti input; Tw output
function Tw = saturation_rw(Lw,Ti)

sat1 = abs(Lw(1))/1.6e-3;
sat2 = abs(Lw(2))/1.6e-3;
sat3 = abs(Lw(3))/1.6e-3;

if sat1>1 && Ti(1)*Lw(1)>0
    T1 = 0;
else 
    T1 = Ti(1);
end

if sat2>1 && Ti(2)*Lw(2)>0
    T2 = 0;
else 
    T2 = Ti(2);
end

if sat3>1 && Ti(3)*Lw(3)>0
    T3 = 0;
else 
    T3 = Ti(3);
end

Tw = [T1;T2;T3];

== matlab function ADCS_Outline/Reaction Wheels Control/MATLAB Function1 ==
  data: mode input; Lwheel input; T output; Nominal input; Calibration input
function T = selector(mode,Lwheel, Nominal, Calibration)

switch mode
    case 6 %Detumbling
        T = -0.5*Lwheel;
    case 7 %OFF
        T = [0;0;0];
    case 8%Calibration
        T = Calibration;
    otherwise
        T = Nominal;
end

== matlab function ADCS_Outline/ITRF to Body/Angle between vectors ==
  data: u input; y output; v input
function y = fcn(u,v)

y = acos(dot(u,v)/(norm(u)*norm(v)))*180/pi;

== matlab function ADCS_Outline/Perfect DCM/Mode Selection ==
  data: DCM_BF input; DCM_BTarget output; Mode input; DCM_S input; DCM_G input; DCM_A input; DCM_N input; DCM_Z input
function DCM_BTarget   = fcn(DCM_BF, Mode,DCM_S,DCM_G, DCM_A, DCM_N, DCM_Z)

switch Mode
    case 1
      DCM_BTarget = DCM_BF*DCM_S;
    case 2
      DCM_BTarget = DCM_BF*DCM_G;
    case 3
      DCM_BTarget = DCM_BF*DCM_A;
    case 4
      DCM_BTarget = DCM_BF*DCM_N;
    case 5
      DCM_BTarget = DCM_BF*DCM_Z;
    otherwise 
      DCM_BTarget = eye(3);
end

== matlab function ADCS_Outline/Guidance&Determination/Guidance/     ==
  data: qa input; q output; qb input
function q = Quatmultiply(qa,qb)

q4 = qa(4)*qb(4) - qa(1)*qb(1) - qa(2)*qb(2) - qa(3)*qb(3);
q1 = qa(4)*qb(1) + qa(1)*qb(4) + qa(2)*qb(3) - qa(3)*qb(2);
q2 = qa(4)*qb(2) - qa(1)*qb(3) + qa(2)*qb(4) + qa(3)*qb(1);
q3 = qa(4)*qb(3) + qa(1)*qb(2) - qa(2)*qb(1) + qa(3)*qb(4);

q = [q1 q2 q3 q4];

== matlab function ADCS_Outline/Toolbox/DCM2W/Anti-Skewed/MATLAB Function ==
  data: u input; y output
function y = fcn(u)
y = [-u(2,3);u(1,3);-u(1,2)];

== matlab function ADCS_Outline/Guidance&Determination/Mode Selection/Mode Selector ==
  data: modeOverdrive input; N input; G input; A input; P input; Eclipse input; Mode output; Ltot input
function Mode  = Selector(modeOverdrive,N, G, A,P,Eclipse,Ltot)

persistent Mode_i
if isempty(Mode_i)
    Mode_i = 7;%OFF
end

switch modeOverdrive
    case 0

        if Mode_i == 6 && norm(Ltot) > 0.9e-3 %bdot exit criteria
           Mode_i = 6; %Detumbling
        elseif max(abs(Ltot)) > 1.7e-3 %saturation
           Mode_i = 6; %Detumbling 
        elseif Eclipse == 1 %twilight
           Mode_i = 5; %Nadir Pointing
        elseif dot(P,A)/(norm(P)*norm(A)) > 0.96 %In range of Argentina
           Mode_i = 3; %Imaging Argentina
        elseif dot(P,N)/(norm(P)*norm(N)) > 0.96 %In range of Namibia
           Mode_i = 4; %Imaging Namibia 
        elseif dot(P,G)/(norm(P)*norm(G)) > 0.91 %In range of ground
           Mode_i = 2; %Ground
        else %default
           Mode_i = 1; %Sun
        end
        
    case 1
           Mode_i = 1; %Sun  
    case 2
           Mode_i = 2; %Ground
    case 3
           Mode_i = 3; %Imaging Argentina
    case 4
           Mode_i = 4; %Imaging Namibia
    case 5
           Mode_i = 5; %Nadir
    case 6
           Mode_i = 6; %Detumbling
    case 8 
           Mode_i = 8; %Calibration
    otherwise
           Mode_i = 7; %OFF
end

Mode = Mode_i;

== matlab function ADCS_Outline/Toolbox/Quat Rot/     ==
  data: qa input; q output; qb input
function q = Quatmultiply(qa,qb)

q4 = qa(4)*qb(4) - qa(1)*qb(1) - qa(2)*qb(2) - qa(3)*qb(3);
q1 = qa(4)*qb(1) + qa(1)*qb(4) + qa(2)*qb(3) - qa(3)*qb(2);
q2 = qa(4)*qb(2) - qa(1)*qb(3) + qa(2)*qb(4) + qa(3)*qb(1);
q3 = qa(4)*qb(3) + qa(1)*qb(2) - qa(2)*qb(1) + qa(3)*qb(4);

q = [q1 q2 q3 q4];

== matlab function ADCS_Outline/Toolbox/MATLAB Function ==
  data: S input; readings output; vectors input
function readings = fcn(S, vectors)

readings = zeros(12,1);

for i=1:1:12

    readings(i) = dot(S,vectors(i,:));
    
    if readings(i)<0
        readings(i) = 0;
    end
    
end

== matlab function ADCS_Outline/Toolbox/Decoder/MATLAB Function1 ==
  data: readings input; A output; vectors input; B output
function [A,B] = fcn(readings, vectors)

[value,pos] = maxk(readings,3);
A = zeros(3);
B = zeros(3,1);

if max(readings)> 0.1 %prevents errors during eclipse
for i = 1:1:3
    A(i,:) = value(i)*vectors(pos(i),:);
    B(i) = (norm(value(i)))^2;
end
else
    A = eye(3);
    B = [0;0;0];
end

%the system is:
%
%  x        y         z
%
% x1        y1        z1      x1^2+y1^2+z1^2
% x2        y2        z2      x2^2+y2^2+z2^2
% x3        y3        z3      x3^2+y3^2+z3^2
%
%where x1 y1 z1 is the reading of one of the sensors in body frame,
%similarly for 2 and 3

== matlab function ADCS_Outline/Toolbox/EKF Test/S//C Kinematics/Skewed/MATLAB Function ==
  data: u input; y output
function y = fcn(u)
y = [ 0     u(3) -u(2) u(1); ...
     -u(3)  0     u(1) u(2); ...
      u(2) -u(1)  0    u(3); ...
     -u(1) -u(2) -u(3) 0];

== matlab function ADCS_Outline/Toolbox/Quat Rot/    1 ==
  data: qa input; q output; qb input
function q = Quatmultiply(qa,qb)

q4 = qa(4)*qb(4) - qa(1)*qb(1) - qa(2)*qb(2) - qa(3)*qb(3);
q1 = qa(4)*qb(1) + qa(1)*qb(4) + qa(2)*qb(3) - qa(3)*qb(2);
q2 = qa(4)*qb(2) - qa(1)*qb(3) + qa(2)*qb(4) + qa(3)*qb(1);
q3 = qa(4)*qb(3) + qa(1)*qb(2) - qa(2)*qb(1) + qa(3)*qb(4);

q = [q1 q2 q3 q4];

== matlab function ADCS_Outline/Toolbox/EKF Test/Quat Rot/     ==
  data: qa input; q output; qb input
function q = Quatmultiply(qa,qb)

q4 = qa(4)*qb(4) - qa(1)*qb(1) - qa(2)*qb(2) - qa(3)*qb(3);
q1 = qa(4)*qb(1) + qa(1)*qb(4) + qa(2)*qb(3) - qa(3)*qb(2);
q2 = qa(4)*qb(2) - qa(1)*qb(3) + qa(2)*qb(4) + qa(3)*qb(1);
q3 = qa(4)*qb(3) + qa(1)*qb(2) - qa(2)*qb(1) + qa(3)*qb(4);

q = [q1 q2 q3 q4];

== matlab function ADCS_Outline/Toolbox/Quat Rot/MATLAB Function ==
  data: u input; y output
function y = fcn(u)

y = [transpose(u) 0];

== matlab function ADCS_Outline/Toolbox/EKF Test/Quat Rot/    1 ==
  data: qa input; q output; qb input
function q = Quatmultiply(qa,qb)

q4 = qa(4)*qb(4) - qa(1)*qb(1) - qa(2)*qb(2) - qa(3)*qb(3);
q1 = qa(4)*qb(1) + qa(1)*qb(4) + qa(2)*qb(3) - qa(3)*qb(2);
q2 = qa(4)*qb(2) - qa(1)*qb(3) + qa(2)*qb(4) + qa(3)*qb(1);
q3 = qa(4)*qb(3) + qa(1)*qb(2) - qa(2)*qb(1) + qa(3)*qb(4);

q = [q1 q2 q3 q4];

== matlab function ADCS_Outline/Toolbox/EKF Test/Quat Rot/MATLAB Function ==
  data: u input; y output
function y = fcn(u)

y = [transpose(u) 0];

== matlab function ADCS_Outline/Toolbox/EKF Test/Quat Rot1/     ==
  data: qa input; q output; qb input
function q = Quatmultiply(qa,qb)

q4 = qa(4)*qb(4) - qa(1)*qb(1) - qa(2)*qb(2) - qa(3)*qb(3);
q1 = qa(4)*qb(1) + qa(1)*qb(4) + qa(2)*qb(3) - qa(3)*qb(2);
q2 = qa(4)*qb(2) - qa(1)*qb(3) + qa(2)*qb(4) + qa(3)*qb(1);
q3 = qa(4)*qb(3) + qa(1)*qb(2) - qa(2)*qb(1) + qa(3)*qb(4);

q = [q1 q2 q3 q4];

== matlab function ADCS_Outline/Toolbox/EKF Test/Quat Rot1/    1 ==
  data: qa input; q output; qb input
function q = Quatmultiply(qa,qb)

q4 = qa(4)*qb(4) - qa(1)*qb(1) - qa(2)*qb(2) - qa(3)*qb(3);
q1 = qa(4)*qb(1) + qa(1)*qb(4) + qa(2)*qb(3) - qa(3)*qb(2);
q2 = qa(4)*qb(2) - qa(1)*qb(3) + qa(2)*qb(4) + qa(3)*qb(1);
q3 = qa(4)*qb(3) + qa(1)*qb(2) - qa(2)*qb(1) + qa(3)*qb(4);

q = [q1 q2 q3 q4];

== matlab function ADCS_Outline/Toolbox/EKF Test/Quat Rot1/MATLAB Function ==
  data: u input; y output
function y = fcn(u)

y = [transpose(u) 0];

== matlab function ADCS_Outline/Toolbox/  ==
  data: dcm input; q output
function q = fcn(dcm)
tr = trace(dcm);

if (tr > 0) 
  S = sqrt(tr+1.0) * 2; % S=4*qw 
  qw = 0.25 * S;
  qx = (dcm(3,2) - dcm(2,3)) / S;
  qy = (dcm(1,3) - dcm(3,1)) / S; 
  qz = (dcm(2,1) - dcm(1,2)) / S; 
elseif ((dcm(1,1) > dcm(2,2)) && (dcm(1,1) > dcm(3,3))) 
  S = sqrt(1.0 + dcm(1,1) - dcm(2,2) - dcm(3,3)) * 2; % S=4*qx 
  qw = (dcm(3,2) - dcm(2,3)) / S;
  qx = 0.25 * S;
  qy = (dcm(1,2) + dcm(2,1)) / S; 
  qz = (dcm(1,3) + dcm(3,1)) / S; 
elseif (dcm(2,2) > dcm(3,3)) 
  S = sqrt(1.0 + dcm(2,2) - dcm(1,1) - dcm(3,3)) * 2; % S=4*qy
  qw = (dcm(1,3) - dcm(3,1)) / S;
  qx = (dcm(1,2) + dcm(2,1)) / S; 
  qy = 0.25 * S;
  qz = (dcm(2,3) + dcm(3,2)) / S; 
 else  
  S = sqrt(1.0 + dcm(3,3) - dcm(1,1) - dcm(2,2)) * 2; % S=4*qz
  qw = (dcm(2,1) - dcm(1,2)) / S;
  qx = (dcm(1,3) + dcm(3,1)) / S;
  qy = (dcm(2,3) + dcm(3,2)) / S;
  qz = 0.25 * S;
end
q = [qx;qy;qz;qw];

== matlab function ADCS_Outline/Guidance&Determination/Body-Earth Estimation/MATLAB Function1 ==
  data: y input; u input; Se input; x output; Be input; I input; step input; Eclipse input; Lw input; P output
function [x,P]    = EKF(y,u,Se,Be,I,step,Eclipse,Lw)

persistent x_check P_check R RE Q invI
%% first guess and Covariance definition 
if isempty(x_check)

    x_check = [triad(Se,Be,y(1:3),y(4:6));0;0;0]; %first guess of state
    P_check = [1.0 0 0 0 0 0 0; %covariance q1 (high guess)
               0 1.0 0 0 0 0 0; %covariance q2
               0 0 1.0 0 0 0 0; %covariance q3
               0 0 0 1.0 0 0 0; %covariance q4
               0 0 0 0 0.1 0 0; %covariance wx
               0 0 0 0 0 0.1 0; %covariance wy
               0 0 0 0 0 0 0.1];%covariance wz
           
    %noise from the sensors     
    R = [1e-4  0 0 0 0 0;  %covariance Sx
         0 1e-4  0 0 0 0;  %covariance Sy
         0 0 1e-4  0 0 0;  %covariance Sz
         0 0 0 2e-14 0 0;  %covariance Bx
         0 0 0 0 2e-14 0;  %covariance By
         0 0 0 0 0 2e-14 ];%covariance Bz
     
    %noise from the sensors in the eclipse
    RE = [2e-14 0 0;  %covariance Bx
          0 2e-14 0;  %covariance By
          0 0 2e-14 ];%covariance Bz
     
    %noise from the prediction 
    Q = [5e-5 0 0 0 0 0 0;... %covariance q1 **FOR STEP TIME OF 0.5s**
         0 5e-5 0 0 0 0 0;... %covariance q2
         0 0 5e-5 0 0 0 0;... %covariance q3
         0 0 0 5e-5 0 0 0;... %covariance q4
         0 0 0 0 2e-8 0 0;... %covariance wx
         0 0 0 0 0 2e-8 0;... %covariance wy
         0 0 0 0 0 0 2e-8];   %covariance wz
     
    invI = inv(I); 
     
end
%% Ports to data
q1 = x_check(1);
q2 = x_check(2);
q3 = x_check(3);
q4 = x_check(4);
wx = x_check(5);
wy = x_check(6);
wz = x_check(7);

% Twx = u(1);
% Twy = u(2);
% Twz = u(3);

hwx = Lw(1);
hwy = Lw(2);
hwz = Lw(3);


%% Prediction
 F = [1 0.5 * step * wz -0.5 * step * wy 0.5 * step * wx 0.5 * step * q4 -0.5 * step * q3 0.5 * step * q2;
     -0.5 * step * wz 1 0.5 * step * wx 0.5 * step * wy 0.5 * step * q3 0.5 * step * q4 -0.5 * step * q1;
     0.5 * step * wy -0.5 * step * wx 1 0.5 * step * wz -0.5 * step * q2 0.5 * step * q1 0.5 * step * q4;
     -0.5 * step * wx -0.5 * step * wy -0.5 * step * wz 1 -0.5 * step * q1 -0.5 * step * q2 -0.5 * step * q3;
     0 0 0 0 step * (invI(1,1) * (wz * I(2,1) - wy * I(3,1)) + invI(1,2) * (-wz * I(1,1) + 2 * I(3,1) * wx + I(3,2) * wy + I(3,3) * wz + hwz) + invI(1,3) * (wy * I(1,1) - 2 * I(2,1) * wx - I(2,2) * wy - I(2,3) * wz - hwy)) + 1 step * (invI(1,1) * (wz * I(2,2) - I(3,1) * wx - 2 * I(3,2) * wy - I(3,3) * wz - hwz) + invI(1,2) * (-wz * I(1,2) + wx * I(3,2)) + invI(1,3) * (I(1,1) * wx + 2 * I(1,2) * wy + I(1,3) * wz - wx * I(2,2) + hwx)) step * (invI(1,1) * (I(2,1) * wx + I(2,2) * wy + 2 * I(2,3) * wz - wy * I(3,3) + hwy) + invI(1,2) * (-I(1,1) * wx - I(1,2) * wy - 2 * I(1,3) * wz + wx * I(3,3) - hwx) + invI(1,3) * (wy * I(1,3) - wx * I(2,3))); 
     0 0 0 0 step * (invI(2,1) * (wz * I(2,1) - wy * I(3,1)) + invI(2,2) * (-wz * I(1,1) + 2 * I(3,1) * wx + I(3,2) * wy + I(3,3) * wz + hwz) + invI(2,3) * (wy * I(1,1) - 2 * I(2,1) * wx - I(2,2) * wy - I(2,3) * wz - hwy)) step * (invI(2,1) * (wz * I(2,2) - I(3,1) * wx - 2 * I(3,2) * wy - I(3,3) * wz - hwz) + invI(2,2) * (-wz * I(1,2) + wx * I(3,2)) + invI(2,3) * (I(1,1) * wx + 2 * I(1,2) * wy + I(1,3) * wz - wx * I(2,2) + hwx)) + 1 step * (invI(2,1) * (I(2,1) * wx + I(2,2) * wy + 2 * I(2,3) * wz - wy * I(3,3) + hwy) + invI(2,2) * (-I(1,1) * wx - I(1,2) * wy - 2 * I(1,3) * wz + wx * I(3,3) - hwx) + invI(2,3) * (wy * I(1,3) - wx * I(2,3)));
     0 0 0 0 step * (invI(3,1) * (wz * I(2,1) - wy * I(3,1)) + invI(3,2) * (-wz * I(1,1) + 2 * I(3,1) * wx + I(3,2) * wy + I(3,3) * wz + hwz) + invI(3,3) * (wy * I(1,1) - 2 * I(2,1) * wx - I(2,2) * wy - I(2,3) * wz - hwy)) step * (invI(3,1) * (wz * I(2,2) - I(3,1) * wx - 2 * I(3,2) * wy - I(3,3) * wz - hwz) + invI(3,2) * (-wz * I(1,2) + wx * I(3,2)) + invI(3,3) * (I(1,1) * wx + 2 * I(1,2) * wy + I(1,3) * wz - wx * I(2,2) + hwx)) step * (invI(3,1) * (I(2,1) * wx + I(2,2) * wy + 2 * I(2,3) * wz - wy * I(3,3) + hwy) + invI(3,2) * (-I(1,1) * wx - I(1,2) * wy - 2 * I(1,3) * wz + wx * I(3,3) - hwx) + invI(3,3) * (wy * I(1,3) - wx * I(2,3))) + 1;];
step=step/10;
for i=1:1:10 
wx = x_check(5);
wy = x_check(6);
wz = x_check(7);

x_check = x_check +[.5*[0  wz -wy wx;
                      -wz  0   wx wy;
                       wy -wx 0   wz;
                      -wx -wy -wz 0]*x_check(1:4)*step;
                      (invI*(cross(-x_check(5:7), I*x_check(5:7)+Lw)-u))*step];%predict state
end
P_check = F*P_check*transpose(F)+Q; %update covariance matrix of state
%% Correction
if Eclipse == 0 %with sun sensors     
    H = [2 * Se(1) * q1 + 2 * Se(2) * q2 + 2 * Se(3) * q3  2 * Se(2) * q1 - 2 * Se(1) * q2 - 2 * Se(3) * q4 2 * Se(3) * q1 - 2 * Se(1) * q3 + 2 * Se(2) * q4 -2 * Se(3) * q2 + 2 * Se(2) * q3 + 2 * Se(1) * q4 0 0 0;
        -2 * Se(2) * q1 + 2 * Se(1) * q2 + 2 * Se(3) * q4  2 * Se(1) * q1 + 2 * Se(2) * q2 + 2 * Se(3) * q3 2 * Se(3) * q2 - 2 * Se(2) * q3 - 2 * Se(1) * q4  2 * Se(3) * q1 - 2 * Se(1) * q3 + 2 * Se(2) * q4 0 0 0;
        -2 * Se(3) * q1 + 2 * Se(1) * q3 - 2 * Se(2) * q4 -2 * Se(3) * q2 + 2 * Se(2) * q3 + 2 * Se(1) * q4 2 * Se(1) * q1 + 2 * Se(2) * q2 + 2 * Se(3) * q3 -2 * Se(2) * q1 + 2 * Se(1) * q2 + 2 * Se(3) * q4 0 0 0;
         2 * Be(1) * q1 + 2 * Be(2) * q2 + 2 * Be(3) * q3  2 * Be(2) * q1 - 2 * Be(1) * q2 - 2 * Be(3) * q4 2 * Be(3) * q1 - 2 * Be(1) * q3 + 2 * Be(2) * q4 -2 * Be(3) * q2 + 2 * Be(2) * q3 + 2 * Be(1) * q4 0 0 0;
        -2 * Be(2) * q1 + 2 * Be(1) * q2 + 2 * Be(3) * q4  2 * Be(1) * q1 + 2 * Be(2) * q2 + 2 * Be(3) * q3 2 * Be(3) * q2 - 2 * Be(2) * q3 - 2 * Be(1) * q4  2 * Be(3) * q1 - 2 * Be(1) * q3 + 2 * Be(2) * q4 0 0 0;
        -2 * Be(3) * q1 + 2 * Be(1) * q3 - 2 * Be(2) * q4 -2 * Be(3) * q2 + 2 * Be(2) * q3 + 2 * Be(1) * q4 2 * Be(1) * q1 + 2 * Be(2) * q2 + 2 * Be(3) * q3 -2 * Be(2) * q1 + 2 * Be(1) * q2 + 2 * Be(3) * q4 0 0 0];

    K = P_check*transpose(H)/((H*P_check*transpose(H)+R));
    x_check = x_check + K*(y-[Quatrot(x_check(1:4).*[-1;-1;-1;1],Se); Quatrot(x_check(1:4).*[-1;-1;-1;1],Be)]);
    P_check = (eye(7)-K*H)*P_check;  

else %no sun sensors in the eclipse 
    HE = [2 * Be(1) * q1 + 2 * Be(2) * q2 + 2 * Be(3) * q3  2 * Be(2) * q1 - 2 * Be(1) * q2 - 2 * Be(3) * q4 2 * Be(3) * q1 - 2 * Be(1) * q3 + 2 * Be(2) * q4 -2 * Be(3) * q2 + 2 * Be(2) * q3 + 2 * Be(1) * q4 0 0 0;
         -2 * Be(2) * q1 + 2 * Be(1) * q2 + 2 * Be(3) * q4  2 * Be(1) * q1 + 2 * Be(2) * q2 + 2 * Be(3) * q3 2 * Be(3) * q2 - 2 * Be(2) * q3 - 2 * Be(1) * q4  2 * Be(3) * q1 - 2 * Be(1) * q3 + 2 * Be(2) * q4 0 0 0;
         -2 * Be(3) * q1 + 2 * Be(1) * q3 - 2 * Be(2) * q4 -2 * Be(3) * q2 + 2 * Be(2) * q3 + 2 * Be(1) * q4 2 * Be(1) * q1 + 2 * Be(2) * q2 + 2 * Be(3) * q3 -2 * Be(2) * q1 + 2 * Be(1) * q2 + 2 * Be(3) * q4 0 0 0];

    K = P_check*transpose(HE)/((HE*P_check*transpose(HE)+RE));
    x_check = x_check + K*(y(4:6)-Quatrot(x_check(1:4).*[-1;-1;-1;1],Be));
    P_check = (eye(7)-K*HE)*P_check;    

end    

x_check(1:4) = x_check(1:4)/norm(x_check(1:4)); %normalise the quaternion
x = x_check.*[-1;-1;-1;1;1;1;1]; %output value     
P = P_check; %output value 

%% functions
function vb = Quatrot(qa,va) %rotate vector by quaternion

q = Quatmultiply(qa,[va;0]);
q = Quatmultiply(q,qa.*[-1;-1;-1;1]); 

vb = q(1:3);

function q = Quatmultiply(qa,qb) %multiply quaternions

q4 = qa(4)*qb(4) - qa(1)*qb(1) - qa(2)*qb(2) - qa(3)*qb(3);
q1 = qa(4)*qb(1) + qa(1)*qb(4) + qa(2)*qb(3) - qa(3)*qb(2);
q2 = qa(4)*qb(2) - qa(1)*qb(3) + qa(2)*qb(4) + qa(3)*qb(1);
q3 = qa(4)*qb(3) + qa(1)*qb(2) - qa(2)*qb(1) + qa(3)*qb(4);

q = [q1;q2;q3;q4]; 

function q_AB = triad(va1,va2,vb1,vb2)

va1=va1/norm(va1);
va2=va2/norm(va2);
vb1=vb1/norm(vb1);
vb2=vb2/norm(vb2);

crossa=cross(va1,va2)/norm(cross(va1,va2));
crossb=cross(vb1,vb2)/norm(cross(vb1,vb2));

DCM_AB=[va1 cross(crossa,va1)/norm(cross(crossa,va1)) crossa]*...
       [vb1 cross(crossb,vb1)/norm(cross(crossb,vb1)) crossb].';
q_AB = DCM2Quat(DCM_AB);
   
function q = DCM2Quat(dcm)
tr = trace(dcm);

if (tr > 0) 
  S = sqrt(tr+1.0) * 2; % S=4*qw 
  qw = 0.25 * S;
  qx = (dcm(3,2) - dcm(2,3)) / S;
  qy = (dcm(1,3) - dcm(3,1)) / S; 
  qz = (dcm(2,1) - dcm(1,2)) / S; 
elseif ((dcm(1,1) > dcm(2,2)) && (dcm(1,1) > dcm(3,3))) 
  S = sqrt(1.0 + dcm(1,1) - dcm(2,2) - dcm(3,3)) * 2; % S=4*qx 
  qw = (dcm(3,2) - dcm(2,3)) / S;
  qx = 0.25 * S;
  qy = (dcm(1,2) + dcm(2,1)) / S; 
  qz = (dcm(1,3) + dcm(3,1)) / S; 
elseif (dcm(2,2) > dcm(3,3)) 
  S = sqrt(1.0 + dcm(2,2) - dcm(1,1) - dcm(3,3)) * 2; % S=4*qy
  qw = (dcm(1,3) - dcm(3,1)) / S;
  qx = (dcm(1,2) + dcm(2,1)) / S; 
  qy = 0.25 * S;
  qz = (dcm(2,3) + dcm(3,2)) / S; 
 else  
  S = sqrt(1.0 + dcm(3,3) - dcm(1,1) - dcm(2,2)) * 2; % S=4*qz
  qw = (dcm(2,1) - dcm(1,2)) / S;
  qx = (dcm(1,3) + dcm(3,1)) / S;
  qy = (dcm(2,3) + dcm(3,2)) / S;
  qz = 0.25 * S;
end
q = [qx;qy;qz;qw];
